simulink model "fsk4_rx"  (R2020b)
settings: Solver=VariableStepAuto  StartTime=0.0  StopTime=2/100e3  RelTol=1e-3
PreLoadFcn:
  | setup_receiver
InitFcn:
  | setup_receiver;
  | fs=100e3;
undefined symbols (not defined in the file): AXI4, Lite
libraries: xbsIndex_r4 x242, hdlsllib x16, commrandsrc3 x2, dsphdlxfrm x1
(part 2 of 2)

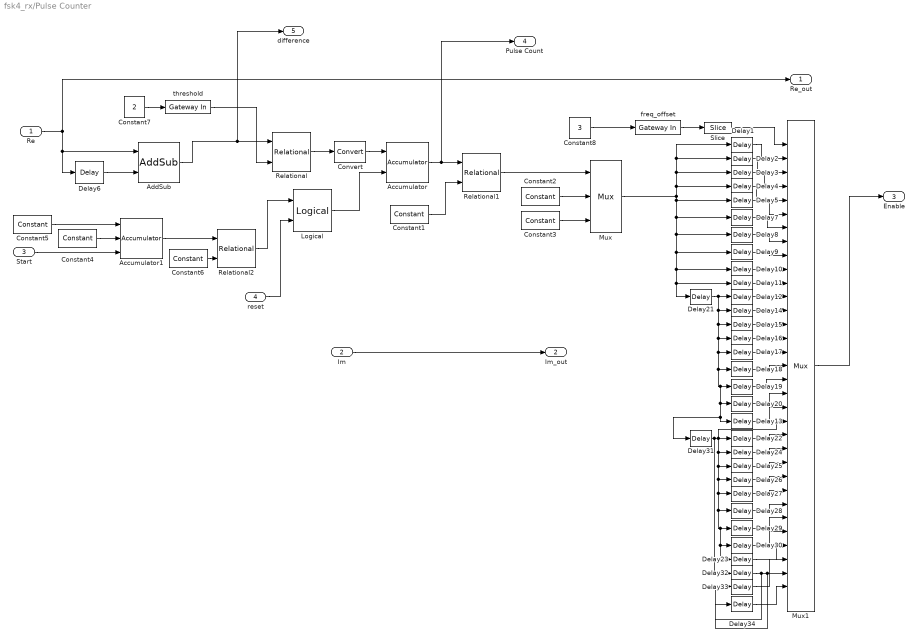
== system fsk4_rx/Pulse Counter ==
  Re : Inport
  Im : Inport  Port=2
  Start : Inport  Port=3
  reset : Inport  Port=4
  Accumulator : xbsIndex_r4/Accumulator  operation=Add  n_bits=16  overflow=Flag as error  scale=1  rst=on  hasbypass=off  infoeditControl=reset for floating point data type must be asserted for a minimum of 2 cycles  en=off  latency=0  msb_inp=100  msb=100  lsb=-100  use_behavioral_HDL=on  implementation=Fabric  dbl_ovrd=off  block_type=accum
  Accumulator1 : xbsIndex_r4/Accumulator  operation=Add  n_bits=16  overflow=Wrap  scale=1  rst=on  hasbypass=off  infoeditControl=reset for floating point data type must be asserted for a minimum of 2 cycles  en=on  latency=0  msb_inp=100  msb=100  lsb=-100  use_behavioral_HDL=on  implementation=Fabric  dbl_ovrd=off  block_type=accum
  AddSub : xbsIndex_r4/AddSub  mode=Subtraction  use_carryin=off  use_carryout=off  en=off  latency=0  precision=User Defined  arith_type="Signed  (2's comp)"  n_bits=16  bin_pt=10  quantization=Truncate  overflow=Wrap  use_behavioral_HDL=off  hw_selection=Fabric  pipelined=off  dbl_ovrd=off  block_type=addsub
  Constant1 : xbsIndex_r4/Constant  const=10  gui_display_data_type=Fixed-point  arith_type=Unsigned  n_bits=16  bin_pt=0  preci_type=Single  exp_width=8  frac_width=24  explicit_period=on  period=1/128e6  equ=P=C  opselect=C  inp2=PCIN>>17  opr=+  inp1=P  carry=CIN  dbl_ovrd=off  block_type=constant
  Constant2 : xbsIndex_r4/Constant  const=0  gui_display_data_type=Boolean  arith_type=Boolean  n_bits=16  bin_pt=14  preci_type=Single  exp_width=8  frac_width=24  explicit_period=on  period=1/128e6  equ=P=C  opselect=C  inp2=PCIN>>17  opr=+  inp1=P  carry=CIN  dbl_ovrd=off  block_type=constant
  Constant3 : xbsIndex_r4/Constant  const=1.0  gui_display_data_type=Boolean  arith_type=Boolean  n_bits=16  bin_pt=14  preci_type=Single  exp_width=8  frac_width=24  explicit_period=on  period=1/128e6  equ=P=C  opselect=C  inp2=PCIN>>17  opr=+  inp1=P  carry=CIN  dbl_ovrd=off  block_type=constant
  Constant4 : xbsIndex_r4/Constant  const=1.0  gui_display_data_type=Boolean  arith_type=Boolean  n_bits=16  bin_pt=14  preci_type=Single  exp_width=8  frac_width=24  explicit_period=on  period=8/128e6  equ=P=C  opselect=C  inp2=PCIN>>17  opr=+  inp1=P  carry=CIN  dbl_ovrd=off  block_type=constant
  Constant5 : xbsIndex_r4/Constant  const=1.0  gui_display_data_type=Fixed-point  arith_type=Unsigned  n_bits=8  bin_pt=0  preci_type=Single  exp_width=8  frac_width=24  explicit_period=on  period=1/128e6  equ=P=C  opselect=C  inp2=PCIN>>17  opr=+  inp1=P  carry=CIN  dbl_ovrd=off  block_type=constant
  Constant6 : xbsIndex_r4/Constant  const=7  gui_display_data_type=Fixed-point  arith_type=Unsigned  n_bits=8  bin_pt=0  preci_type=Single  exp_width=8  frac_width=24  explicit_period=on  period=1/128e6  equ=P=C  opselect=C  inp2=PCIN>>17  opr=+  inp1=P  carry=CIN  dbl_ovrd=off  block_type=constant
  Constant7 : Constant  Value=2  OutDataTypeStr=fixdt(1,16,14)
  Constant8 : Constant  Value=3  OutDataTypeStr=fixdt(1,16,12)
  Convert : xbsIndex_r4/Convert  gui_display_data_type=Fixed-point  arith_type=Unsigned  n_bits=8  bin_pt=0  float_type=Single  exp_bits=8  fraction_bits=24  quantization=Truncate  overflow=Wrap  en=off  latency=0  pipeline=off  dbl_ovrd=off  block_type=convert
  Delay{1,6,12,22,33} (5 alike) : xbsIndex_r4/Delay  rst=off  infoeditControl=Selection of Reset will increase slice count due to use of real FFs and instead of SRLs  en=off  latency=1  reg_retiming=off  dbl_ovrd=off  block_type=delay
  Delay10 : xbsIndex_r4/Delay  rst=off  infoeditControl=Selection of Reset will increase slice count due to use of real FFs and instead of SRLs  en=off  latency=9  reg_retiming=off  dbl_ovrd=off  block_type=delay
  Delay{11,21,31..32} (4 alike) : xbsIndex_r4/Delay  rst=off  infoeditControl=Selection of Reset will increase slice count due to use of real FFs and instead of SRLs  en=off  latency=10  reg_retiming=off  dbl_ovrd=off  block_type=delay
  Delay13 : xbsIndex_r4/Delay  rst=off  infoeditControl=Selection of Reset will increase slice count due to use of real FFs and instead of SRLs  en=off  latency=9  reg_retiming=off  dbl_ovrd=off  block_type=delay
  Delay{2,14,24,34} (4 alike) : xbsIndex_r4/Delay  rst=off  infoeditControl=Selection of Reset will increase slice count due to use of real FFs and instead of SRLs  en=off  latency=2  reg_retiming=off  dbl_ovrd=off  block_type=delay
  Delay15 : xbsIndex_r4/Delay  rst=off  infoeditControl=Selection of Reset will increase slice count due to use of real FFs and instead of SRLs  en=off  latency=3  reg_retiming=off  dbl_ovrd=off  block_type=delay
  Delay16 : xbsIndex_r4/Delay  rst=off  infoeditControl=Selection of Reset will increase slice count due to use of real FFs and instead of SRLs  en=off  latency=4  reg_retiming=off  dbl_ovrd=off  block_type=delay
  Delay17 : xbsIndex_r4/Delay  rst=off  infoeditControl=Selection of Reset will increase slice count due to use of real FFs and instead of SRLs  en=off  latency=5  reg_retiming=off  dbl_ovrd=off  block_type=delay
  Delay18 : xbsIndex_r4/Delay  rst=off  infoeditControl=Selection of Reset will increase slice count due to use of real FFs and instead of SRLs  en=off  latency=6  reg_retiming=off  dbl_ovrd=off  block_type=delay
  Delay19 : xbsIndex_r4/Delay  rst=off  infoeditControl=Selection of Reset will increase slice count due to use of real FFs and instead of SRLs  en=off  latency=7  reg_retiming=off  dbl_ovrd=off  block_type=delay
  Delay20 : xbsIndex_r4/Delay  rst=off  infoeditControl=Selection of Reset will increase slice count due to use of real FFs and instead of SRLs  en=off  latency=8  reg_retiming=off  dbl_ovrd=off  block_type=delay
  Delay23 : xbsIndex_r4/Delay  rst=off  infoeditControl=Selection of Reset will increase slice count due to use of real FFs and instead of SRLs  en=off  latency=9  reg_retiming=off  dbl_ovrd=off  block_type=delay
  Delay25 : xbsIndex_r4/Delay  rst=off  infoeditControl=Selection of Reset will increase slice count due to use of real FFs and instead of SRLs  en=off  latency=3  reg_retiming=off  dbl_ovrd=off  block_type=delay
  Delay26 : xbsIndex_r4/Delay  rst=off  infoeditControl=Selection of Reset will increase slice count due to use of real FFs and instead of SRLs  en=off  latency=4  reg_retiming=off  dbl_ovrd=off  block_type=delay
  Delay27 : xbsIndex_r4/Delay  rst=off  infoeditControl=Selection of Reset will increase slice count due to use of real FFs and instead of SRLs  en=off  latency=5  reg_retiming=off  dbl_ovrd=off  block_type=delay
  Delay28 : xbsIndex_r4/Delay  rst=off  infoeditControl=Selection of Reset will increase slice count due to use of real FFs and instead of SRLs  en=off  latency=6  reg_retiming=off  dbl_ovrd=off  block_type=delay
  Delay29 : xbsIndex_r4/Delay  rst=off  infoeditControl=Selection of Reset will increase slice count due to use of real FFs and instead of SRLs  en=off  latency=7  reg_retiming=off  dbl_ovrd=off  block_type=delay
  Delay3 : xbsIndex_r4/Delay  rst=off  infoeditControl=Selection of Reset will increase slice count due to use of real FFs and instead of SRLs  en=off  latency=3  reg_retiming=off  dbl_ovrd=off  block_type=delay
  Delay30 : xbsIndex_r4/Delay  rst=off  infoeditControl=Selection of Reset will increase slice count due to use of real FFs and instead of SRLs  en=off  latency=8  reg_retiming=off  dbl_ovrd=off  block_type=delay
  Delay4 : xbsIndex_r4/Delay  rst=off  infoeditControl=Selection of Reset will increase slice count due to use of real FFs and instead of SRLs  en=off  latency=4  reg_retiming=off  dbl_ovrd=off  block_type=delay
  Delay5 : xbsIndex_r4/Delay  rst=off  infoeditControl=Selection of Reset will increase slice count due to use of real FFs and instead of SRLs  en=off  latency=5  reg_retiming=off  dbl_ovrd=off  block_type=delay
  Delay7 : xbsIndex_r4/Delay  rst=off  infoeditControl=Selection of Reset will increase slice count due to use of real FFs and instead of SRLs  en=off  latency=6  reg_retiming=off  dbl_ovrd=off  block_type=delay
  Delay8 : xbsIndex_r4/Delay  rst=off  infoeditControl=Selection of Reset will increase slice count due to use of real FFs and instead of SRLs  en=off  latency=7  reg_retiming=off  dbl_ovrd=off  block_type=delay
  Delay9 : xbsIndex_r4/Delay  rst=off  infoeditControl=Selection of Reset will increase slice count due to use of real FFs and instead of SRLs  en=off  latency=8  reg_retiming=off  dbl_ovrd=off  block_type=delay
  Logical : xbsIndex_r4/Logical  logical_function=OR  inputs=2  en=off  latency=0  precision=Full  arith_type=Unsigned  n_bits=16  bin_pt=0  align_bp=on  dbl_ovrd=off  block_type=logical
  Mux : xbsIndex_r4/Mux  inputs=2  en=off  latency=0  precision=Full  arith_type=Unsigned  n_bits=16  bin_pt=14  quantization=Truncate  overflow=Wrap  dbl_ovrd=off  block_type=mux
  Mux1 : xbsIndex_r4/Mux  inputs=32  en=off  latency=0  precision=Full  arith_type=Unsigned  n_bits=16  bin_pt=14  quantization=Truncate  overflow=Wrap  dbl_ovrd=off  block_type=mux
  Relational : xbsIndex_r4/Relational  mode=a>b  op_type=Bool  en=off  latency=0  dbl_ovrd=off  block_type=relational
  Relational1 : xbsIndex_r4/Relational  mode=a=b  op_type=Bool  en=off  latency=0  dbl_ovrd=off  block_type=relational
  Relational2 : xbsIndex_r4/Relational  mode=a=b  op_type=Bool  en=off  latency=0  dbl_ovrd=off  block_type=relational
  Slice : xbsIndex_r4/Slice  nbits=1  boolean_output=off  mode=Two Bit Locations  bit1=4  base1=LSB of Input  bit0=0  base0=LSB of Input  dbl_ovrd=off  block_type=slice
  freq_offset : xbsIndex_r4/Gateway In  gui_display_data_type=Fixed-point  arith_type=Unsigned  n_bits=8  bin_pt=0  preci_type=Single  exp_width=8  frac_width=24  rows=1  columns=1  quantization="Round  (unbiased: +/- Inf)"  overflow=Saturate  period=1/128e6  UseAsADC=off  ADCChannel='1'  interface=AXI4-Lite  automatic_assignment=off  address_offset=40  intf_name=''  intf_description=''  default_value=3  timing_constraint=None  locs_specified=off  LOCs={}  io_standard={}  inherit_from_input=off  hdl_port=on  dbl_ovrd=off  block_type=gatewayin
  threshold : xbsIndex_r4/Gateway In  gui_display_data_type=Fixed-point  arith_type="Signed  (2's comp)"  n_bits=16  bin_pt=14  preci_type=Single  exp_width=8  frac_width=24  rows=1  columns=1  quantization="Round  (unbiased: +/- Inf)"  overflow=Saturate  period=1/128e6  UseAsADC=off  ADCChannel='1'  interface=AXI4-Lite  automatic_assignment=off  address_offset=12  intf_name=''  intf_description=''  default_value=0.4  timing_constraint=None  locs_specified=off  LOCs={}  io_standard={}  inherit_from_input=off  hdl_port=on  dbl_ovrd=off  block_type=gatewayin
  Re_out : Outport
  Im_out : Outport  Port=2
  Enable : Outport  Port=3
  Pulse Count : Outport  Port=4
  difference : Outport  Port=5
  wires:
  Im/1 -> Im_out/1
  Delay6/1 -> AddSub/2
  Constant1/1 -> Relational1/2
  Constant3/1 -> Mux/3
  Constant2/1 -> Mux/2
  Relational1/1 -> Mux/1
  Convert/1 -> Accumulator/1
  Relational/1 -> Convert/1
  Constant4/1 -> Accumulator1/2
  Start/1 -> Accumulator1/3
  Constant5/1 -> Accumulator1/1
  Accumulator1/1 -> Relational2/1
  Constant6/1 -> Relational2/2
  Relational2/1 -> Logical/1
  Accumulator/1 -> Pulse Count/1, Relational1/1
  Re/1 -> Re_out/1, AddSub/1, Delay6/1
  Constant7/1 -> threshold/1
  threshold/1 -> Relational/2
  Logical/1 -> Accumulator/2
  AddSub/1 -> difference/1, Relational/1
  Mux1/1 -> Enable/1
  Delay1/1 -> Mux1/2
  Delay2/1 -> Mux1/3
  Delay3/1 -> Mux1/4
  Delay4/1 -> Mux1/5
  Delay5/1 -> Mux1/6
  Delay7/1 -> Mux1/7
  Delay8/1 -> Mux1/8
  Delay9/1 -> Mux1/9
  Mux/1 -> Delay4/1, Delay3/1, Delay2/1, Delay1/1, Delay10/1, Delay11/1, Delay21/1, Delay9/1, Delay8/1, Delay7/1, Delay5/1
  freq_offset/1 -> Slice/1
  Constant8/1 -> freq_offset/1
  Slice/1 -> Mux1/1
  Delay10/1 -> Mux1/10
  Delay11/1 -> Mux1/11
  Delay12/1 -> Mux1/12
  Delay14/1 -> Mux1/13
  Delay15/1 -> Mux1/14
  Delay16/1 -> Mux1/15
  Delay17/1 -> Mux1/16
  Delay18/1 -> Mux1/17
  Delay19/1 -> Mux1/18
  Delay20/1 -> Mux1/19
  Delay13/1 -> Mux1/20
  Delay21/1 -> Delay31/1, Delay13/1, Delay20/1, Delay19/1, Delay18/1, Delay17/1, Delay16/1, Delay15/1, Delay14/1, Delay12/1
  Delay31/1 -> Delay32/1, Delay23/1, Delay30/1, Delay29/1, Delay28/1, Delay27/1, Delay26/1, Delay25/1, Delay24/1, Delay22/1, Mux1/21
  Delay22/1 -> Mux1/22
  Delay24/1 -> Mux1/23
  Delay25/1 -> Mux1/24
  Delay26/1 -> Mux1/25
  Delay27/1 -> Mux1/26
  Delay28/1 -> Mux1/27
  Delay29/1 -> Mux1/28
  Delay30/1 -> Mux1/29
  Delay23/1 -> Mux1/30
  Delay32/1 -> Delay34/1, Mux1/31, Delay33/1
  Delay33/1 -> Mux1/32
  Delay34/1 -> Mux1/33
  reset/1 -> Logical/2

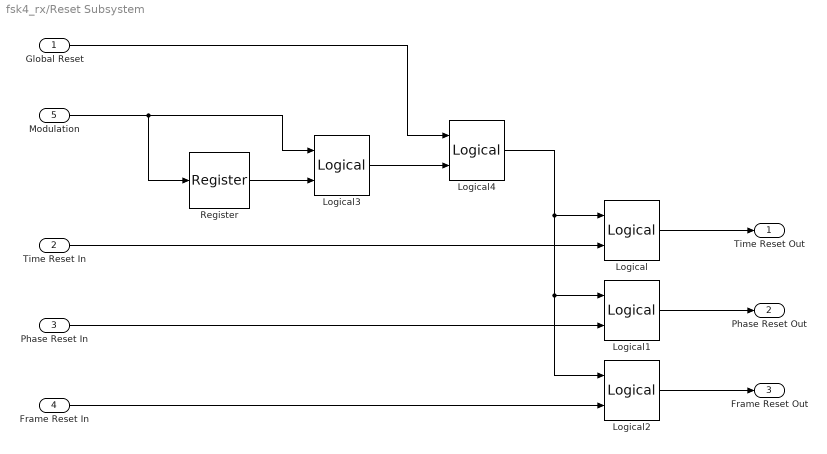
== system fsk4_rx/Reset Subsystem ==
  Global Reset : Inport
  Time Reset In : Inport  Port=2
  Phase Reset In : Inport  Port=3
  Frame Reset In : Inport  Port=4
  Modulation : Inport  Port=5
  Logical{,1..2,4} (4 alike) : xbsIndex_r4/Logical  logical_function=OR  inputs=2  en=off  latency=0  precision=Full  arith_type=Unsigned  n_bits=16  bin_pt=0  align_bp=on  dbl_ovrd=off  block_type=logical
  Logical3 : xbsIndex_r4/Logical  logical_function=XOR  inputs=2  en=off  latency=0  precision=Full  arith_type=Unsigned  n_bits=16  bin_pt=0  align_bp=on  dbl_ovrd=off  block_type=logical
  Register : xbsIndex_r4/Register  init=0  rst=off  en=off  dbl_ovrd=off  block_type=register
  Time Reset Out : Outport
  Phase Reset Out : Outport  Port=2
  Frame Reset Out : Outport  Port=3
  wires:
  Time Reset In/1 -> Logical/2
  Logical/1 -> Time Reset Out/1
  Phase Reset In/1 -> Logical1/2
  Frame Reset In/1 -> Logical2/2
  Logical2/1 -> Frame Reset Out/1
  Logical1/1 -> Phase Reset Out/1
  Modulation/1 -> Logical3/1, Register/1
  Global Reset/1 -> Logical4/1
  Logical4/1 -> Logical2/1, Logical1/1, Logical/1
  Register/1 -> Logical3/2
  Logical3/1 -> Logical4/2

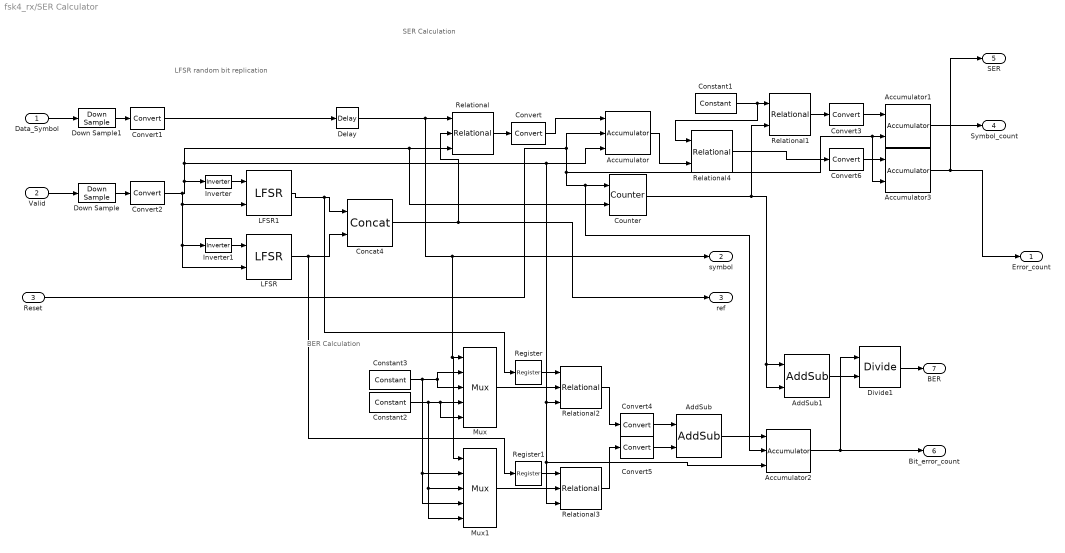
== system fsk4_rx/SER Calculator ==
  note: LFSR random bit replication
  note: BER Calculation
  note: SER Calculation
  Data_Symbol : Inport
  Valid : Inport  Port=2
  Reset : Inport  Port=3
  Accumulator : xbsIndex_r4/Accumulator  operation=Add  n_bits=32  overflow=Wrap  scale=1  rst=on  hasbypass=off  infoeditControl=reset for floating point data type must be asserted for a minimum of 2 cycles  en=on  latency=1  msb_inp=100  msb=100  lsb=-100  use_behavioral_HDL=on  implementation=Fabric  dbl_ovrd=off  block_type=accum
  Accumulator1 : xbsIndex_r4/Accumulator  operation=Add  n_bits=16  overflow=Wrap  scale=1  rst=on  hasbypass=off  infoeditControl=reset for floating point data type must be asserted for a minimum of 2 cycles  en=off  latency=1  msb_inp=100  msb=100  lsb=-100  use_behavioral_HDL=on  implementation=Fabric  dbl_ovrd=off  block_type=accum
  Accumulator2 : xbsIndex_r4/Accumulator  operation=Add  n_bits=8  overflow=Wrap  scale=1  rst=on  hasbypass=off  infoeditControl=reset for floating point data type must be asserted for a minimum of 2 cycles  en=on  latency=1  msb_inp=100  msb=100  lsb=-100  use_behavioral_HDL=on  implementation=Fabric  dbl_ovrd=off  block_type=accum
  Accumulator3 : xbsIndex_r4/Accumulator  operation=Add  n_bits=16  overflow=Wrap  scale=1  rst=on  hasbypass=off  infoeditControl=reset for floating point data type must be asserted for a minimum of 2 cycles  en=off  latency=1  msb_inp=100  msb=100  lsb=-100  use_behavioral_HDL=on  implementation=Fabric  dbl_ovrd=off  block_type=accum
  AddSub : xbsIndex_r4/AddSub  mode=Addition  use_carryin=off  use_carryout=off  en=off  latency=0  precision=Full  arith_type=Unsigned  n_bits=16  bin_pt=14  quantization=Truncate  overflow=Wrap  use_behavioral_HDL=off  hw_selection=Fabric  pipelined=off  dbl_ovrd=off  block_type=addsub
  AddSub1 : xbsIndex_r4/AddSub  mode=Addition  use_carryin=off  use_carryout=off  en=off  latency=0  precision=Full  arith_type=Unsigned  n_bits=16  bin_pt=14  quantization=Truncate  overflow=Wrap  use_behavioral_HDL=off  hw_selection=Fabric  pipelined=off  dbl_ovrd=off  block_type=addsub
  Concat4 : xbsIndex_r4/Concat  num_inputs=2  dbl_ovrd=off  block_type=concat
  Constant1 : xbsIndex_r4/Constant  const=4e6  gui_display_data_type=Fixed-point  arith_type=Unsigned  n_bits=32  bin_pt=0  preci_type=Single  exp_width=8  frac_width=24  explicit_period=on  period=1/4e6  equ=P=C  opselect=C  inp2=PCIN>>17  opr=+  inp1=P  carry=CIN  dbl_ovrd=off  block_type=constant
  Constant2 : xbsIndex_r4/Constant  const=1  gui_display_data_type=Fixed-point  arith_type=Unsigned  n_bits=1  bin_pt=0  preci_type=Single  exp_width=8  frac_width=24  explicit_period=on  period=1/4e6  equ=P=C  opselect=C  inp2=PCIN>>17  opr=+  inp1=P  carry=CIN  dbl_ovrd=off  block_type=constant
  Constant3 : xbsIndex_r4/Constant  const=0  gui_display_data_type=Fixed-point  arith_type=Unsigned  n_bits=1  bin_pt=0  preci_type=Single  exp_width=8  frac_width=24  explicit_period=on  period=1/4e6  equ=P=C  opselect=C  inp2=PCIN>>17  opr=+  inp1=P  carry=CIN  dbl_ovrd=off  block_type=constant
  Convert{,3..6} (5 alike) : xbsIndex_r4/Convert  gui_display_data_type=Fixed-point  arith_type=Unsigned  n_bits=1  bin_pt=0  float_type=Single  exp_bits=8  fraction_bits=24  quantization=Truncate  overflow=Wrap  en=off  latency=0  pipeline=off  dbl_ovrd=off  block_type=convert
  Convert1 : xbsIndex_r4/Convert  gui_display_data_type=Fixed-point  arith_type=Unsigned  n_bits=2  bin_pt=0  float_type=Single  exp_bits=8  fraction_bits=24  quantization=Truncate  overflow=Wrap  en=off  latency=0  pipeline=off  dbl_ovrd=off  block_type=convert
  Convert2 : xbsIndex_r4/Convert  gui_display_data_type=Boolean  arith_type=Boolean  n_bits=2  bin_pt=0  float_type=Single  exp_bits=8  fraction_bits=24  quantization=Truncate  overflow=Wrap  en=off  latency=0  pipeline=off  dbl_ovrd=off  block_type=convert
  Counter : xbsIndex_r4/Counter  cnt_type=Count Limited  cnt_to=4e6  operation=Up  start_count=1  cnt_by_val=1  arith_type=Unsigned  n_bits=32  bin_pt=0  load_pin=off  rst=on  en=on  explicit_period=on  period=1/4e6  use_behavioral_HDL=off  implementation=Fabric  dbl_ovrd=off  block_type=counter
  Delay : xbsIndex_r4/Delay  rst=off  infoeditControl=Selection of Reset will increase slice count due to use of real FFs and instead of SRLs  en=off  latency=2  reg_retiming=off  dbl_ovrd=off  block_type=delay
  Divide1 : xbsIndex_r4/Divide  flow_control=NonBlocking  axi_optimize_goal=Resources  algorithm_type=Radix2  infoedit1=Specify output fraction-width for Fixed-point division.  fractional_width=32  infoedit2=Specify latency for Floating-point division.  latency=1  rate=1  has_a_tlast=off  has_a_tuser=off  has_b_tlast=off  has_b_tuser=off  en=off  has_result_tready=off  result_tlast_behv=Pass_A_TLAST  has_underflow=off  has_overflow=off  has_invalid_op=off  has_divide_by_zero=off  fpo_op_type=mergeddivide  block_type=divide
      settings: infoedit=Blocking: Wait for data on all inputs, allow back-pressure.<br>NonBlocking: operate every cycle in which all inputs are valid, no back-pressure.
  Down Sample : xbsIndex_r4/Down Sample  sample_ratio=32  sample_phase="Last Value of Frame  (most efficient)"  en=off  rst=off  latency=1  dbl_ovrd=off  block_type=dsamp
  Down Sample1 : xbsIndex_r4/Down Sample  sample_ratio=32  sample_phase="Last Value of Frame  (most efficient)"  en=off  rst=off  latency=1  dbl_ovrd=off  block_type=dsamp
  Inverter : xbsIndex_r4/Inverter  en=off  latency=0  dbl_ovrd=off  block_type=inv
  Inverter1 : xbsIndex_r4/Inverter  en=off  latency=0  dbl_ovrd=off  block_type=inv
  LFSR : xbsIndex_r4/LFSR  lfsr_type=Fibonacci  gate_type=XNOR  n_bits=10  maxpolynomial=on  polynomial='121'  rst_value='000'  rst=on  en=on  reloadable_seed=off  input_type=off  output_type=off  arith_type="Signed  (2's comp)"  bin_pt=4  explicit_period=on  period=1/4e6  dbl_ovrd=off  block_type=lfsr
  LFSR1 : xbsIndex_r4/LFSR  lfsr_type=Fibonacci  gate_type=XNOR  n_bits=16  maxpolynomial=on  polynomial='6805'  rst_value='0000'  rst=on  en=on  reloadable_seed=off  input_type=off  output_type=off  arith_type="Signed  (2's comp)"  bin_pt=4  explicit_period=on  period=1/4e6  dbl_ovrd=off  block_type=lfsr
  Mux : xbsIndex_r4/Mux  inputs=4  en=off  latency=1  precision=Full  arith_type=Unsigned  n_bits=16  bin_pt=14  quantization=Truncate  overflow=Wrap  dbl_ovrd=off  block_type=mux
  Mux1 : xbsIndex_r4/Mux  inputs=4  en=off  latency=1  precision=Full  arith_type=Unsigned  n_bits=16  bin_pt=14  quantization=Truncate  overflow=Wrap  dbl_ovrd=off  block_type=mux
  Register : xbsIndex_r4/Register  init=0  rst=off  en=off  dbl_ovrd=off  block_type=register
  Register1 : xbsIndex_r4/Register  init=0  rst=off  en=off  dbl_ovrd=off  block_type=register
  Relational : xbsIndex_r4/Relational  mode=a!=b  op_type=Bool  en=on  latency=1  dbl_ovrd=off  block_type=relational
  Relational1 : xbsIndex_r4/Relational  mode=a=b  op_type=Bool  en=off  latency=1  dbl_ovrd=off  block_type=relational
  Relational2 : xbsIndex_r4/Relational  mode=a!=b  op_type=Bool  en=on  latency=1  dbl_ovrd=off  block_type=relational
  Relational3 : xbsIndex_r4/Relational  mode=a!=b  op_type=Bool  en=on  latency=1  dbl_ovrd=off  block_type=relational
  Relational4 : xbsIndex_r4/Relational  mode=a=b  op_type=Bool  en=off  latency=1  dbl_ovrd=off  block_type=relational
  Error_count : Outport
  symbol : Outport  Port=2
  ref : Outport  Port=3
  Symbol_count : Outport  Port=4
  SER : Outport  Port=5
  Bit_error_count : Outport  Port=6
  BER : Outport  Port=7
  wires:
  LFSR/1 -> Register1/1, Concat4/2
  LFSR1/1 -> Register/1, Concat4/1
  Relational/1 -> Convert/1
  Convert/1 -> Accumulator/1
  Convert1/1 -> Delay/1
  Data_Symbol/1 -> Down Sample1/1
  Valid/1 -> Down Sample/1
  Down Sample/1 -> Convert2/1
  Down Sample1/1 -> Convert1/1
  Concat4/1 -> ref/1, Relational/2
  Delay/1 -> symbol/1, Mux1/1, Mux/1, Relational/1
  Inverter/1 -> LFSR1/1
  Convert2/1 -> Inverter1/1, LFSR/2, LFSR1/2, Relational2/3, Relational3/3, Accumulator2/3, Accumulator/3, Counter/2, Relational/3, Inverter/1
  Inverter1/1 -> LFSR/1
  Convert3/1 -> Accumulator1/1
  Accumulator/1 -> Relational4/2
  Constant1/1 -> Relational4/1, Relational1/1
  Counter/1 -> AddSub1/2, AddSub1/1, Relational1/2
  Reset/1 -> Counter/1, Accumulator2/2, Accumulator3/2, Accumulator1/2, Accumulator/2
  Relational1/1 -> Convert3/1
  Accumulator1/1 -> Symbol_count/1
  Constant2/1 -> Mux1/5, Mux1/3, Mux/4, Mux/5
  Constant3/1 -> Mux1/4, Mux1/2, Mux/3, Mux/2
  Mux/1 -> Relational2/2
  Register/1 -> Relational2/1
  Mux1/1 -> Relational3/2
  Register1/1 -> Relational3/1
  Relational2/1 -> Convert4/1
  Relational3/1 -> Convert5/1
  Convert4/1 -> AddSub/1
  Convert5/1 -> AddSub/2
  AddSub/1 -> Accumulator2/1
  Accumulator2/1 -> Divide1/1, Bit_error_count/1
  AddSub1/1 -> Divide1/2
  Divide1/1 -> BER/1
  Convert6/1 -> Accumulator3/1
  Relational4/1 -> Convert6/1
  Accumulator3/1 -> SER/1, Error_count/1

== system fsk4_rx/AXI-Stream Master Interface/Rising Edge Detector Enable ==
  Input : Inport
  Inverter2 : xbsIndex_r4/Inverter  en=off  latency=0  dbl_ovrd=off  block_type=inv
  Logical3 : xbsIndex_r4/Logical  logical_function=AND  inputs=2  en=off  latency=0  precision=Full  arith_type=Unsigned  n_bits=16  bin_pt=0  align_bp=on  dbl_ovrd=off  block_type=logical
  Register1 : xbsIndex_r4/Register  init=0  rst=off  en=off  dbl_ovrd=off  block_type=register
  Output : Outport  VectorParamsAs1DForOutWhenUnconnected=off
  wires:
  Input/1 -> Logical3/2, Inverter2/1
  Inverter2/1 -> Register1/1
  Logical3/1 -> Output/1
  Register1/1 -> Logical3/1

== system fsk4_rx/AXI-Stream Master Interface/Rising Edge Detector Last ==
  Input : Inport
  Inverter2 : xbsIndex_r4/Inverter  en=off  latency=0  dbl_ovrd=off  block_type=inv
  Logical3 : xbsIndex_r4/Logical  logical_function=AND  inputs=2  en=off  latency=0  precision=Full  arith_type=Unsigned  n_bits=16  bin_pt=0  align_bp=on  dbl_ovrd=off  block_type=logical
  Register1 : xbsIndex_r4/Register  init=0  rst=off  en=off  dbl_ovrd=off  block_type=register
  Output : Outport  VectorParamsAs1DForOutWhenUnconnected=off
  wires:
  Register1/1 -> Logical3/1
  Logical3/1 -> Output/1
  Inverter2/1 -> Register1/1
  Input/1 -> Inverter2/1, Logical3/2

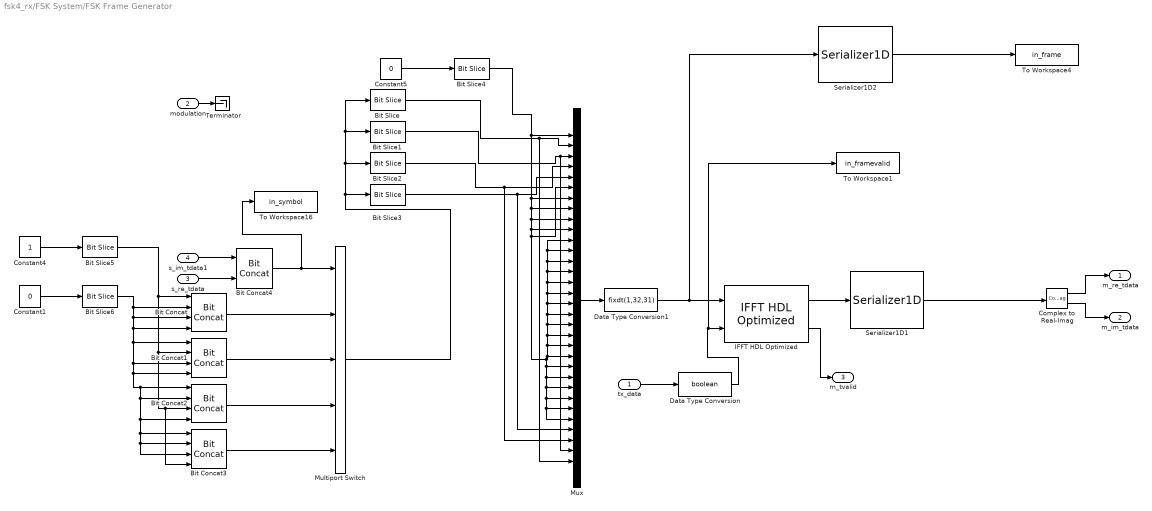
== system fsk4_rx/FSK System/FSK Frame Generator ==
  tx_data : Inport
  modulation : Inport  Port=2
  s_re_tdata : Inport  Port=3
  s_im_tdata1 : Inport  Port=4
  Bit Concat{,1..3} (4 alike) : hdlsllib/Logic and Bit Operations/Bit Concat  numInputs=4
  Bit Concat4 : hdlsllib/Logic and Bit Operations/Bit Concat  numInputs=2
  Bit Slice : hdlsllib/Logic and Bit Operations/Bit Slice  lidx=3  ridx=3
      settings: SourceProductBaseCode=SL
  Bit Slice1 : hdlsllib/Logic and Bit Operations/Bit Slice  lidx=2  ridx=2
      settings: SourceProductBaseCode=SL
  Bit Slice2 : hdlsllib/Logic and Bit Operations/Bit Slice  lidx=1  ridx=1
      settings: SourceProductBaseCode=SL
  Bit Slice{3..6} (4 alike) : hdlsllib/Logic and Bit Operations/Bit Slice  lidx=0  ridx=0
      settings: SourceProductBaseCode=SL
  Complex to Real-Imag : ComplexToRealImag
  Constant1 : Constant  Value=0  OutDataTypeStr=boolean  SampleTime=32/128e6
  Constant4 : Constant  OutDataTypeStr=boolean  SampleTime=32/128e6
  Constant5 : Constant  Value=0  OutDataTypeStr=boolean  SampleTime=32/128e6
  Data Type Conversion : DataTypeConversion  OutDataTypeStr=boolean
  Data Type Conversion1 : DataTypeConversion  OutDataTypeStr=fixdt(1,32,31)
  IFFT HDL Optimized : dsphdlxfrm/IFFT HDL Optimized  FFTLength=32  Architecture=Streaming Radix 2^2  ComplexMultiplication=Use 4 multipliers and 2 adders  BitReversedOutput=off  BitReversedInput=off  Normalize=off  SimulateUsing=Code generation  RoundingMethod=Floor  ResetInputPort=off  StartOutputPort=off  EndOutputPort=off
      settings: SourceProductBaseCode=DS
  Multiport Switch : MultiPortSwitch  DataPortOrder=Zero-based contiguous  Inputs=4  zeroidx=on
  Mux : Mux  Inputs=32
  Serializer1D1 : hdlsllib/HDL Operations/Serializer1D  Ratio=32  IdleCycles=0  validIn=off  startOut=off  validOut=off  inputDataDimensions=-1  inputSampleTime=-1  inputSignalType=auto
      settings: SourceProductBaseCode=SL
  Serializer1D2 : hdlsllib/HDL Operations/Serializer1D  Ratio=32  IdleCycles=0  validIn=off  startOut=off  validOut=off  inputDataDimensions=-1  inputSampleTime=-1  inputSignalType=auto
      settings: SourceProductBaseCode=SL
  Terminator : Terminator
  To Workspace1 : ToWorkspace  VariableName=in_framevalid  SaveFormat=Timeseries  SampleTime=-1
  To Workspace16 : ToWorkspace  VariableName=in_symbol  SaveFormat=Timeseries  SampleTime=-1
  To Workspace4 : ToWorkspace  VariableName=in_frame  SaveFormat=Timeseries  SampleTime=-1
  m_re_tdata : Outport
  m_im_tdata : Outport  Port=2
  m_tvalid : Outport  Port=3
  wires:
  modulation/1 -> Terminator/1
  s_im_tdata1/1 -> Bit Concat4/1
  s_re_tdata/1 -> Bit Concat4/2
  Constant4/1 -> Bit Slice5/1
  Constant1/1 -> Bit Slice6/1
  Bit Concat4/1 -> To Workspace16/1, Multiport Switch/1
  tx_data/1 -> Data Type Conversion/1
  Complex to Real-Imag/1 -> m_re_tdata/1
  Complex to Real-Imag/2 -> m_im_tdata/1
  IFFT HDL Optimized/2 -> m_tvalid/1
  Data Type Conversion/1 -> To Workspace1/1, IFFT HDL Optimized/2
  Constant5/1 -> Bit Slice4/1
  Bit Concat/1 -> Multiport Switch/2
  Bit Concat1/1 -> Multiport Switch/3
  Bit Concat2/1 -> Multiport Switch/4
  Bit Concat3/1 -> Multiport Switch/5
  Multiport Switch/1 -> Bit Slice/1, Bit Slice1/1, Bit Slice2/1, Bit Slice3/1
  Bit Slice/1 -> Mux/2, Mux/32
  Bit Slice1/1 -> Mux/31, Mux/3
  Bit Slice2/1 -> Mux/30, Mux/4
  Bit Slice3/1 -> Mux/29, Mux/5
  Bit Slice4/1 -> Mux/1, Mux/23, Mux/24, Mux/25, Mux/26, Mux/27, Mux/28, Mux/21, Mux/20, Mux/19, Mux/18, Mux/17, Mux/16, Mux/15, Mux/14, Mux/13, Mux/12, Mux/11, Mux/22, Mux/6, Mux/10, Mux/9, Mux/8, Mux/7
  Bit Slice5/1 -> Bit Concat/1, Bit Concat1/2, Bit Concat3/4, Bit Concat2/3
  Bit Slice6/1 -> Bit Concat/2, Bit Concat/3, Bit Concat/4, Bit Concat1/1, Bit Concat1/3, Bit Concat1/4, Bit Concat2/1, Bit Concat2/2, Bit Concat2/4, Bit Concat3/1, Bit Concat3/2, Bit Concat3/3
  IFFT HDL Optimized/1 -> Serializer1D1/1
  Data Type Conversion1/1 -> Serializer1D2/1, IFFT HDL Optimized/1
  Mux/1 -> Data Type Conversion1/1
  Serializer1D1/1 -> Complex to Real-Imag/1
  Serializer1D2/1 -> To Workspace4/1

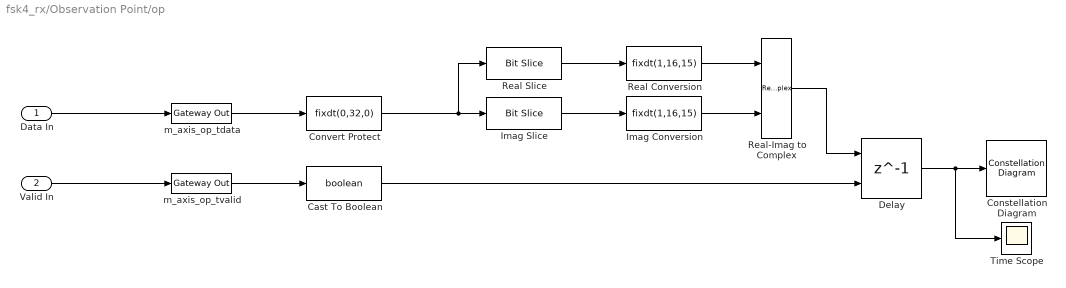
== system fsk4_rx/Observation Point/op ==
  Data In : Inport
  Valid In : Inport  Port=2
  Cast To Boolean : DataTypeConversion  OutDataTypeStr=boolean
  Constellation Diagram : ConstellationDiagram
  Convert Protect : DataTypeConversion  OutDataTypeStr=fixdt(0,32,0)  ConvertRealWorld=Stored Integer (SI)
  Delay : Delay  DelayLength=1  ShowEnablePort=on
      settings: InputPortMap=u0,e6
  Imag Conversion : DataTypeConversion  OutDataTypeStr=fixdt(1,16,15)  ConvertRealWorld=Stored Integer (SI)
  Imag Slice : hdlsllib/Logic and Bit Operations/Bit Slice  lidx=31  ridx=16
      settings: SourceProductBaseCode=SL
  Real Conversion : DataTypeConversion  OutDataTypeStr=fixdt(1,16,15)  ConvertRealWorld=Stored Integer (SI)
  Real Slice : hdlsllib/Logic and Bit Operations/Bit Slice  lidx=15  ridx=0
      settings: SourceProductBaseCode=SL
  Real-Imag to Complex : RealImagToComplex
  Time Scope : Scope
  m_axis_op_tdata : xbsIndex_r4/Gateway Out  inherit_from_input=on  hdl_port=on  rows=1  columns=1  UseAsDAC=off  DACChannel='1'  interface=None  automatic_assignment=on  address_offset=hex2dec('00')  intf_name=''  intf_description=''  timing_constraint=None  locs_specified=off  LOCs={}  io_standard={}  block_type=gatewayout
  m_axis_op_tvalid : xbsIndex_r4/Gateway Out  inherit_from_input=on  hdl_port=on  rows=1  columns=1  UseAsDAC=off  DACChannel='1'  interface=None  automatic_assignment=on  address_offset=hex2dec('00')  intf_name=''  intf_description=''  timing_constraint=None  locs_specified=off  LOCs={}  io_standard={}  block_type=gatewayout
  wires:
  Cast To Boolean/1 -> Delay/2
  Convert Protect/1 -> Imag Slice/1, Real Slice/1
  Real-Imag to Complex/1 -> Delay/1
  m_axis_op_tdata/1 -> Convert Protect/1
  Imag Conversion/1 -> Real-Imag to Complex/2
  Imag Slice/1 -> Imag Conversion/1
  Real Slice/1 -> Real Conversion/1
  Real Conversion/1 -> Real-Imag to Complex/1
  m_axis_op_tvalid/1 -> Cast To Boolean/1
  Delay/1 -> Constellation Diagram/1, Time Scope/1
  Data In/1 -> m_axis_op_tdata/1
  Valid In/1 -> m_axis_op_tvalid/1
